simulink model "Ldqp"  (R2019b)
settings: Solver=ode4  StartTime=0.0  StopTime=1  FixedStep=1e-4  RelTol=1e-3
values from neighbouring files (symbols this model uses):
  Dec = 1    [Sotfware_Matlab.m]
  Lpu = X_ind/ Lb    [Sotfware_Matlab.m]
  Rpu = R_ind / Zb    [Sotfware_Matlab.m]
  w1pu = 1    [Sotfware_Matlab.m]
  wb = Frecuencia_Red*2*pi    (= 314.159265359)    [Sotfware_Matlab.m]
settings Model: Creator=aurelio  LastModifiedBy=jorge
settings DataIOCC: ReturnWorkspaceOutputs=off
settings DebuggingCC: PregeneratedLibrarySubsystemCodeDiagnostic=none  ArithmeticOperatorsInVariantConditions=warning
settings SFSimCC: SimUseLocalCustomCode=off  CustomCodeUndefinedFunction=UseInterfaceOnly
settings RTWCC: RTWUseLocalCustomCode=off
settings CodeAppCC: StateflowObjectComments=on

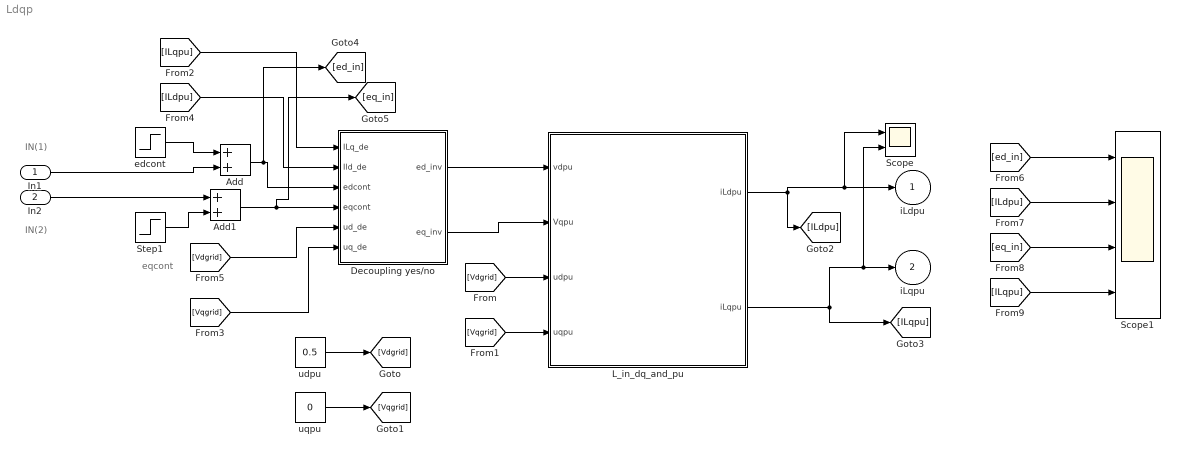
== system Ldqp ==
  note: IN(2)
  note: IN(1)
  note: eqcont
  In1 : Inport
  In2 : Inport  Port=2
  Add : Sum
  Add1 : Sum
  Decoupling yes/no : Subsystem
  L_in_dq_and_pu : Subsystem
  Scope : Scope  NumInputPorts=2
  Scope1 : Scope  NumInputPorts=4
  Step1 : Step  Time=0.8  After=0.5  SampleTime=0
  edcont : Step  Time=0.3  After=0.5  SampleTime=0
  udpu : Constant  Value=0.5
  uqpu : Constant  Value=0
  iLdpu : Outport  VectorParamsAs1DForOutWhenUnconnected=off
  iLqpu : Outport  Port=2  VectorParamsAs1DForOutWhenUnconnected=off
  wires:
  L_in_dq_and_pu/2(iLqpu) -> [ILqpu], Scope/2, iLqpu/1
  L_in_dq_and_pu/1(iLdpu) -> [ILdpu], Scope/1, iLdpu/1
  udpu/1 -> [Vdgrid]
  uqpu/1 -> [Vqgrid]
  [Vdgrid] -> L_in_dq_and_pu/3(udpu)
  [Vqgrid] -> L_in_dq_and_pu/4(uqpu)
  [ILqpu] -> Decoupling yes/no/1(ILq_de)
  [ILdpu] -> Decoupling yes/no/2(Ild_de)
  [Vdgrid] -> Decoupling yes/no/5(ud_de)
  [Vqgrid] -> Decoupling yes/no/6(uq_de)
  Decoupling yes/no/1(ed_inv) -> L_in_dq_and_pu/1(vdpu)
  Decoupling yes/no/2(eq_inv) -> L_in_dq_and_pu/2(Vqpu)
  [ed_in] -> Scope1/1
  [ILdpu] -> Scope1/2
  [eq_in] -> Scope1/3
  [ILqpu] -> Scope1/4
  In1/1 -> Add/2
  edcont/1 -> Add/1
  Step1/1 -> Add1/2
  In2/1 -> Add1/1
  Add/1 -> [ed_in], Decoupling yes/no/3(edcont)
  Add1/1 -> [eq_in], Decoupling yes/no/4(eqcont)

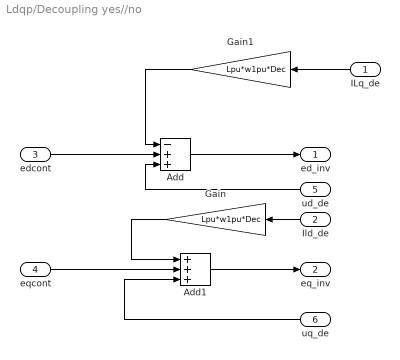
== system Ldqp/Decoupling yes//no ==
  ILq_de : Inport
  Ild_de : Inport  Port=2
  edcont : Inport  Port=3
  eqcont : Inport  Port=4
  ud_de : Inport  Port=5
  uq_de : Inport  Port=6
  Add : Sum  Inputs=-++
  Add1 : Sum  Inputs=+++
  Gain : Gain  Gain=Lpu*w1pu*Dec
  Gain1 : Gain  Gain=Lpu*w1pu*Dec
  ed_inv : Outport  VectorParamsAs1DForOutWhenUnconnected=off
  eq_inv : Outport  Port=2  VectorParamsAs1DForOutWhenUnconnected=off
  wires:
  Add1/1 -> eq_inv/1
  ILq_de/1 -> Gain1/1
  eqcont/1 -> Add1/2
  Gain1/1 -> Add/1
  Ild_de/1 -> Gain/1
  Gain/1 -> Add1/1
  Add/1 -> ed_inv/1
  edcont/1 -> Add/2
  ud_de/1 -> Add/3
  uq_de/1 -> Add1/3

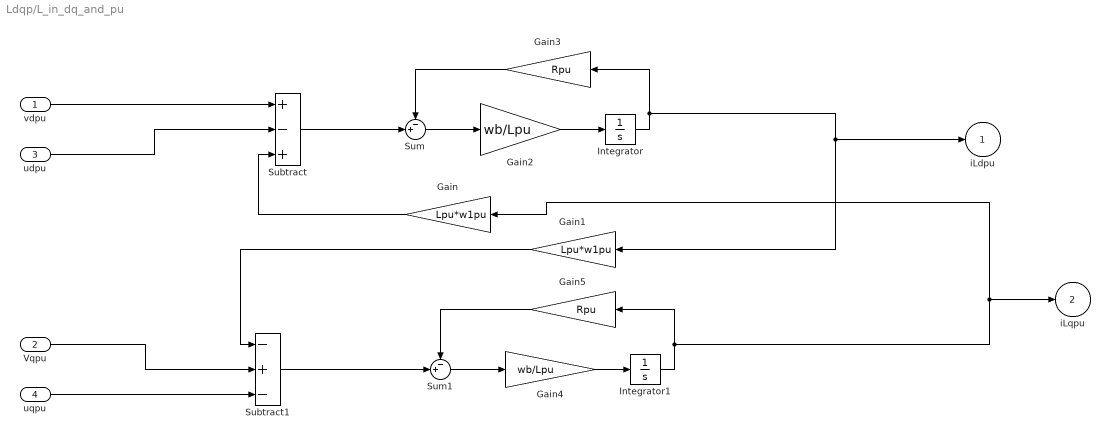
== system Ldqp/L_in_dq_and_pu ==
  vdpu : Inport
  Vqpu : Inport  Port=2
  udpu : Inport  Port=3
  uqpu : Inport  Port=4
  Gain : Gain  Gain=Lpu*w1pu
  Gain1 : Gain  Gain=Lpu*w1pu
  Gain2 : Gain  Gain=wb/Lpu
  Gain3 : Gain  Gain=Rpu
  Gain4 : Gain  Gain=wb/Lpu
  Gain5 : Gain  Gain=Rpu
  Integrator : Integrator
  Integrator1 : Integrator
  Subtract : Sum  Inputs=+-+
  Subtract1 : Sum  Inputs=-+-
  Sum : Sum  Inputs=-+|
  Sum1 : Sum  Inputs=-+|
  iLdpu : Outport  VectorParamsAs1DForOutWhenUnconnected=off
  iLqpu : Outport  Port=2  VectorParamsAs1DForOutWhenUnconnected=off
  wires:
  vdpu/1 -> Subtract/1
  Integrator/1 -> iLdpu/1, Gain1/1, Gain3/1
  Gain/1 -> Subtract/3
  Gain1/1 -> Subtract1/1
  Integrator1/1 -> iLqpu/1, Gain/1, Gain5/1
  Gain2/1 -> Integrator/1
  uqpu/1 -> Subtract1/3
  udpu/1 -> Subtract/2
  Subtract/1 -> Sum/2
  Sum/1 -> Gain2/1
  Gain3/1 -> Sum/1
  Sum1/1 -> Gain4/1
  Gain4/1 -> Integrator1/1
  Gain5/1 -> Sum1/1
  Subtract1/1 -> Sum1/2
  Vqpu/1 -> Subtract1/2
